simulink model "CNcell"  (R2016b)
settings: Solver=ode1  StartTime=0.0  StopTime=5000  FixedStep=0.1  RelTol=1e-3  EnableMultiTasking=on
model workspace: external: MAT-File CN.mat (data not in the file)
values from neighbouring files (symbols this model uses):
  h = gca    [Plottrace.m]    (also in plotCells.m; plotCells_second.m)
  m = m+1    (= 1)    [plotCells.m]    (also in plotCells_second.m)
  s = [4 8 9 10 11]    [plotCells.m]    (also in plotCells_second.m)
undefined symbols (not defined in the file or in its folder): bcl, erp, f, hr, hs, j, r, Vh
libraries: Libs x1
settings Model: PauseTimes=18000  Creator=wai484  LastModifiedBy=wai484
settings DataIOCC: LimitDataPoints=on  SaveFormat=Array
settings OptimizationCC: LifeSpan=inf
settings DebuggingCC: SolverPrmCheckMsg=warning  SFUnexpectedBacktrackingDiag=warning  SFNoUnconditionalDefaultTransitionDiag=warning  SFExecutionAtInitializationDiag=none
settings HardwareCC: ProdBitPerPointer=32  ProdBitPerSizeT=32  ProdBitPerPtrDiffT=32  ProdLargestAtomicFloat=None  ProdIntDivRoundTo=Undefined  ProdEndianess=Unspecified  ProdWordSize=32  ProdHWDeviceType=32-bit Generic
settings ModelReferenceCC: PropagateSignalLabelsOutOfModel=off
settings GRTTargetCC: TargetLangStandard=C89/C90 (ANSI)  GeneratePreprocessorConditionals=Disable all
settings ConfigComp: CovMetricSettings=dw  CovHtmlReporting=on  CovSaveCumulativeToWorkspaceVar=on  CovSaveSingleToWorkspaceVar=on  CovExternalEMLEnable=off  CovSFcnEnable=off

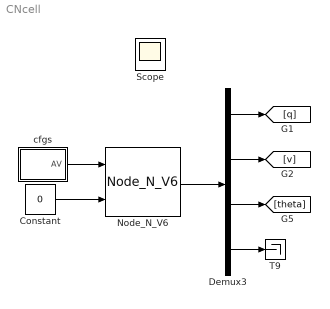
== system CNcell ==
  Constant : Constant  Value=0
  Demux3 : Demux  Outputs=[1, 1, 1,2]
  Node_N_V6 : Libs/Node_N_V6
  T9 : Terminator
  cfgs : Stateflow chart  TreatAsAtomicUnit=on
  Scope : Scope
  wires:
  Node_N_V6/1 -> Demux3/1
  Demux3/4 -> T9/1
  Demux3/1 -> [q]
  Demux3/2 -> [v]
  Demux3/3 -> [theta]
  Constant/1 -> Node_N_V6/2
  cfgs/1(AV) -> Node_N_V6/1

== stateflow chart CNcell/cfgs ==
  settings: executeAtInitialization=1
  state Ini
  (default) -> Ini : {AV=auto;}
  data: erp parameter; Vh parameter; hr parameter; hs parameter; m parameter; s parameter; j parameter; h parameter; f parameter; r parameter; bcl parameter; cfg function_output; AV output
  function cfg = auto:
    | function cfg = auto
    | 
    | BCL=bcl;
    | SD=2;
    | f1=0.1;
    | f2=0.25;
    | sigma1sq=0.0035;
    | sigma2sq=0.007;
    | 
    | d2=3.34; %av
    | erp_out=erp;
    | d0=-0.9448; %av
    | MDP=-74.65; %av
    | VT=25.05; %av
    | VR=41.25; %av
    | Vh_out=Vh;
    | 
    | hr_out=hr; 
    | hs_out=hs;
    | s_out=s;
    | j_out=j;
    | m_out=m; 
    | 
    | h_out=h;
    | f_out=f;
    | 
    | r_out=r;
    | 
    | x=135.5;
    | y=295.5;
    | 
    | cfg=[BCL, SD, f1,f2,sigma1sq, sigma2sq,d2,erp_out,d0,MDP,VT,VR,Vh_out,hr_out,hs_out,s_out,j_out,m_out,h_out,f_out,r_out,x,y];
    | 
    | end
